simulink model "model_Quadrotor6_NonAdaptiveV2"  (R2024b)
settings: Solver=FixedStepAuto  StartTime=0.0  StopTime=T  FixedStep=0.0005  RelTol=1e-3
values from neighbouring files (symbols this model uses):
  ap1_hat = Dp/(kFF*dF*kVF^2)    (= 50.695107696)    [run_Quadrotor6_NonAdaptiveV2.m]
  ap2_hat = m*g*dcm/(kFF*dF*kVF^2)    (= 222.324678221)    [run_Quadrotor6_NonAdaptiveV2.m]
  ap3_hat = -kRT1/(kFF*dF*kVF^2)    (= -0.071301136)    [run_Quadrotor6_NonAdaptiveV2.m]
  ap4_hat = -kRT2/(kFF*dF*kVF^2)    (= -0.0008912642)    [run_Quadrotor6_NonAdaptiveV2.m]
  ay1_hat = -Dy/(kRF*dR*kVR^2)    (= -156.8624992)    [run_Quadrotor6_NonAdaptiveV2.m]
  ay2_hat = kFT1/(kRF*dR*kVR^2)    (= 0.071301136)    [run_Quadrotor6_NonAdaptiveV2.m]
  ay3_hat = kFT2/(kRF*dR*kVR^2)    (= 0.0008912642)    [run_Quadrotor6_NonAdaptiveV2.m]
  control_gains = [lambda_p lambda_y ... (first row only)    [run_Quadrotor6_NonAdaptiveV2.m]
  hp_hat = Jp/(kFF*dF*kVF^2)    (= 156.14948784)    [run_Quadrotor6_NonAdaptiveV2.m]
  hy_hat = -Jy/(kRF*dR*kVR^2)    (= -263.8142032)    [run_Quadrotor6_NonAdaptiveV2.m]
  mtr_select = 0    [run_Quadrotor6_NonAdaptiveV2.m]
  params_haaaa = [hp_hat hy_hat ... (first row only)    [run_Quadrotor6_NonAdaptiveV2.m]
settings Model: Creator=ryanmathewson  LastModifiedBy=samue
settings DebuggingCC: UnconnectedInputMsg=warning  UnconnectedOutputMsg=warning  UnconnectedLineMsg=warning
settings ModelReferenceCC: EnableRefExpFcnMdlSchedulingChecks=on
settings RTWCC: GPUComputeCapability=3.5  DLArmComputeVersion=19.05

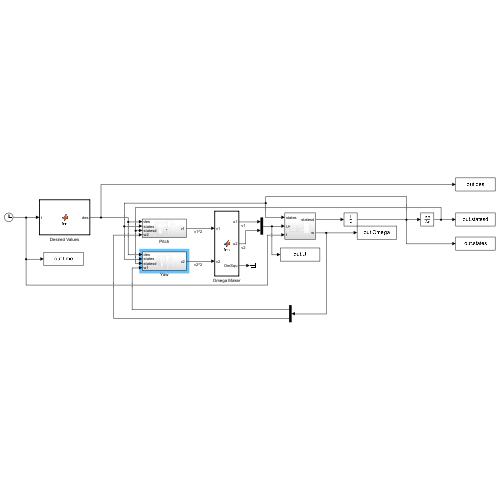
[thumbnail: Simulink's stored preview of the top-level diagram]
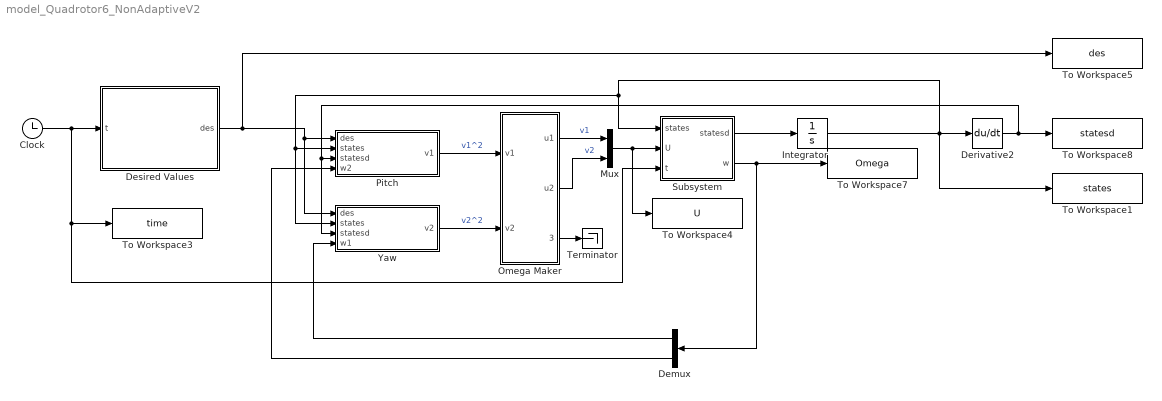
== system model_Quadrotor6_NonAdaptiveV2 ==
  Clock : Clock
  Demux : Demux  Outputs=2
  Derivative2 : Derivative
  Desired Values : MATLAB Function  TreatAsAtomicUnit=on
  Integrator : Integrator  InitialCondition=[0;0;0;0]
  Mux : Mux  Inputs=2
  Omega Maker : MATLAB Function  TreatAsAtomicUnit=on
  Pitch : Subsystem
  Subsystem : Subsystem
  Terminator : Terminator
  To Workspace1 : ToWorkspace  VariableName=states  SampleTime=-1
  To Workspace3 : ToWorkspace  VariableName=time  SampleTime=-1
  To Workspace4 : ToWorkspace  VariableName=U  SampleTime=-1
  To Workspace5 : ToWorkspace  VariableName=des  SampleTime=-1
  To Workspace7 : ToWorkspace  VariableName=Omega  SampleTime=-1
  To Workspace8 : ToWorkspace  VariableName=statesd  SampleTime=-1
  Yaw : Subsystem
  wires:
  Clock/1 -> Subsystem/3(t), To Workspace3/1, Desired Values/1(t)
  Desired Values/1(des) -> To Workspace5/1, Yaw/1(des), Pitch/1(des)
  Pitch/1(v1) -> Omega Maker/1(v1)  "v1^2"
  Yaw/1(v2) -> Omega Maker/2(v2)  "v2^2"
  Omega Maker/1(u1) -> Mux/1  "v1"
  Integrator/1 -> Derivative2/1, Yaw/2(states), Pitch/2(states), Subsystem/1(states), To Workspace1/1
  Subsystem/1(statesd) -> Integrator/1
  Derivative2/1 -> Yaw/3(statesd), Pitch/3(statesd), To Workspace8/1
  Mux/1 -> To Workspace4/1, Subsystem/2(U)
  Omega Maker/2(u2) -> Mux/2  "v2"
  Omega Maker/3(OmSqu) -> Terminator/1
  Subsystem/2(w) -> Demux/1, To Workspace7/1
  Demux/1 -> Yaw/4(w1)
  Demux/2 -> Pitch/4(w2)

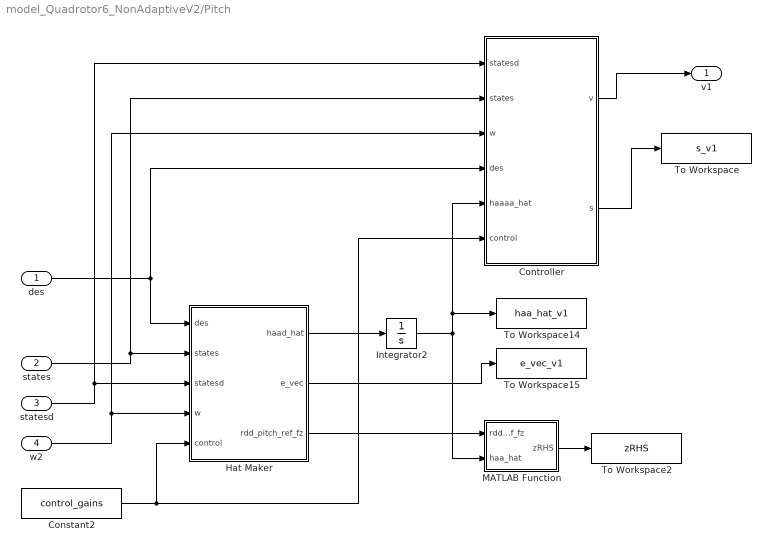
== system model_Quadrotor6_NonAdaptiveV2/Pitch ==
  des : Inport
  states : Inport  Port=2
  statesd : Inport  Port=3
  w2 : Inport  Port=4
  Constant2 : Constant  Value=control_gains
  Controller : MATLAB Function  TreatAsAtomicUnit=on
  Hat Maker : MATLAB Function  TreatAsAtomicUnit=on
  Integrator2 : Integrator  InitialCondition=[hp_hat;ap1_hat;ap2_hat;ap3_hat;ap4_hat]
  MATLAB Function : MATLAB Function  TreatAsAtomicUnit=on
  To Workspace : ToWorkspace  VariableName=s_v1  SampleTime=-1
  To Workspace14 : ToWorkspace  VariableName=haa_hat_v1  SampleTime=-1
  To Workspace15 : ToWorkspace  VariableName=e_vec_v1  SampleTime=-1
  To Workspace2 : ToWorkspace  VariableName=zRHS  SampleTime=-1
  v1 : Outport
  wires:
  Integrator2/1 -> To Workspace14/1, Controller/5(haaaa_hat), MATLAB Function/2(haa_hat)
  Hat Maker/1(haad_hat) -> Integrator2/1
  Hat Maker/2(e_vec) -> To Workspace15/1
  Controller/1(v) -> v1/1
  states/1 -> Controller/2(states), Hat Maker/2(states)
  Controller/2(s) -> To Workspace/1
  des/1 -> Hat Maker/1(des), Controller/4(des)
  statesd/1 -> Controller/1(statesd), Hat Maker/3(statesd)
  MATLAB Function/1(zRHS) -> To Workspace2/1
  Hat Maker/3(rdd_pitch_ref_fz) -> MATLAB Function/1(rdd_ref_fz)
  w2/1 -> Hat Maker/4(w), Controller/3(w)
  Constant2/1 -> Hat Maker/5(control), Controller/6(control)

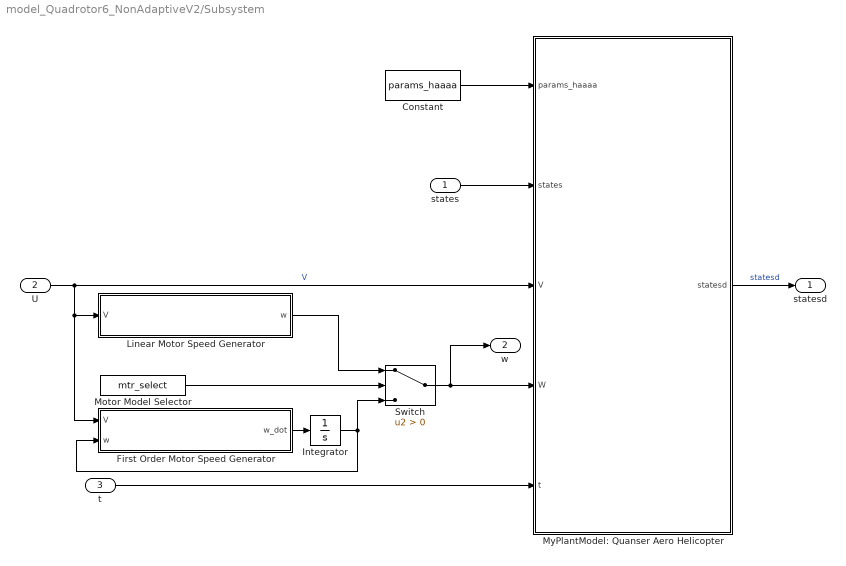
== system model_Quadrotor6_NonAdaptiveV2/Subsystem ==
  states : Inport  PortDimensions=[4 1]
  U : Inport  Port=2  PortDimensions=[2 1]
  t : Inport  Port=3
  Constant : Constant  Value=params_haaaa
  First Order Motor Speed Generator : MATLAB Function  TreatAsAtomicUnit=on
  Integrator : Integrator  InitialCondition=[0;0]
  Linear Motor Speed Generator : MATLAB Function  TreatAsAtomicUnit=on
  Motor Model Selector : Constant  Value=mtr_select
  MyPlantModel: Quanser Aero Helicopter : MATLAB Function  TreatAsAtomicUnit=on
  Switch : Switch  Criteria=u2 > Threshold  SaturateOnIntegerOverflow=off  InputSameDT=off
  statesd : Outport  PortDimensions=[4 1]
  w : Outport  Port=2  PortDimensions=[2 1]
  wires:
  states/1 -> MyPlantModel: Quanser Aero Helicopter/2(states)
  U/1 -> First Order Motor Speed Generator/1(V), Linear Motor Speed Generator/1(V), MyPlantModel: Quanser Aero Helicopter/3(V)  "V"
  t/1 -> MyPlantModel: Quanser Aero Helicopter/5(t)
  MyPlantModel: Quanser Aero Helicopter/1(statesd) -> statesd/1  "statesd"
  First Order Motor Speed Generator/1(w_dot) -> Integrator/1
  Integrator/1 -> Switch/3, First Order Motor Speed Generator/2(w)
  Constant/1 -> MyPlantModel: Quanser Aero Helicopter/1(params_haaaa)
  Switch/1 -> w/1, MyPlantModel: Quanser Aero Helicopter/4(W)
  Linear Motor Speed Generator/1(w) -> Switch/1
  Motor Model Selector/1 -> Switch/2

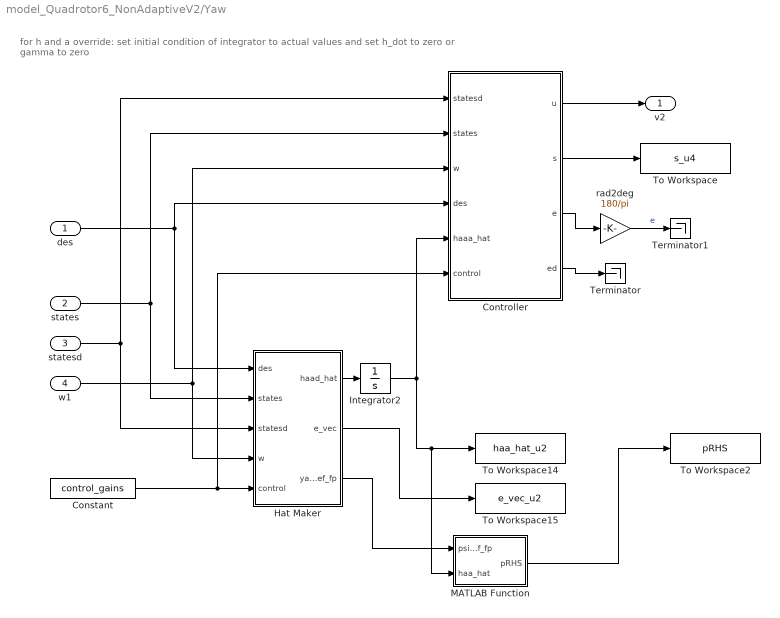
== system model_Quadrotor6_NonAdaptiveV2/Yaw ==
  note: for h and a override: set initial condition of integrator to actual values and set h_dot to zero or gamma to zero
  des : Inport
  states : Inport  Port=2
  statesd : Inport  Port=3
  w1 : Inport  Port=4
  Constant : Constant  Value=control_gains
  Controller : MATLAB Function  TreatAsAtomicUnit=on
  Hat Maker : MATLAB Function  TreatAsAtomicUnit=on
  Integrator2 : Integrator  InitialCondition=[hy_hat;ay1_hat;ay2_hat;ay3_hat]
  MATLAB Function : MATLAB Function  TreatAsAtomicUnit=on
  Terminator : Terminator
  Terminator1 : Terminator
  To Workspace : ToWorkspace  VariableName=s_u4  SampleTime=-1
  To Workspace14 : ToWorkspace  VariableName=haa_hat_u2  SampleTime=-1
  To Workspace15 : ToWorkspace  VariableName=e_vec_u2  SampleTime=-1
  To Workspace2 : ToWorkspace  VariableName=pRHS  SampleTime=-1
  rad2deg : Gain  Gain=180/pi
  v2 : Outport
  wires:
  Integrator2/1 -> Controller/5(haaa_hat), MATLAB Function/2(haa_hat), To Workspace14/1
  des/1 -> Hat Maker/1(des), Controller/4(des)
  Hat Maker/2(e_vec) -> To Workspace15/1
  Hat Maker/1(haad_hat) -> Integrator2/1
  Controller/1(u) -> v2/1
  Controller/2(s) -> To Workspace/1
  states/1 -> Controller/2(states), Hat Maker/2(states)
  statesd/1 -> Controller/1(statesd), Hat Maker/3(statesd)
  MATLAB Function/1(pRHS) -> To Workspace2/1
  Hat Maker/3(yawdd_ref_fp) -> MATLAB Function/1(psidd_ref_fp)
  w1/1 -> Hat Maker/4(w), Controller/3(w)
  Controller/3(e) -> rad2deg/1
  Controller/4(ed) -> Terminator/1
  rad2deg/1 -> Terminator1/1  "e"
  Constant/1 -> Controller/6(control), Hat Maker/5(control)

== matlab function model_Quadrotor6_NonAdaptiveV2/Yaw/Hat Maker ==
  data: des input; states input; haad_hat output; e_vec output; statesd input; yawdd_ref_fp output; w input; control input
function [haad_hat,e_vec,yawdd_ref_fp] = fcn(des,states,statesd, w, control)
%% initialize outputs
haad_hat = zeros(4,1);
e_vec = zeros(2,1);
yawdd_ref_fp = zeros(4,1);

%% separate input vectors
r_yaw = states(2,1);
r_omega_f = w;

rd_yaw = statesd(2,1);

yaw_des = des(4,1);
yawd_des = des(5,1);
yawdd_des = des(6,1);

%% parameters

gamma_0 = 0;
gamma_1 = 0;
gamma_2 = 0;
gamma_3 = 0;

lambda = control(1,2);
D = control(2,2);
eta = control(3,2);
phi_para = control(4,2);
%phi = (abs(a1v_tilde*yd + a2v_tilde*y)+eta)/(h_hat+k);

%% functions
e = r_yaw-yaw_des;
ed = rd_yaw-yawd_des;
yawdd_ref = -(-yawdd_des + lambda*ed) ; %2*lambda*ed + lambda^2*e;
s = ed + lambda*e;

%saturation function
if s>phi_para
  sat = 1;
elseif (s>=-phi_para)&&(s<=phi_para)
  sat = s/phi_para;
else
  sat = -1;
end

s_delta = s - (phi_para * sat);

f1 = rd_yaw;
f2 = r_omega_f;
f3 = sign(r_omega_f)*r_omega_f^2;

%% outputs
hd_hat  = gamma_0^2 * s_delta * (yawdd_ref + ((D + eta) * sat));
a1d_hat = -gamma_1^2 * s_delta * f1;
a2d_hat = -gamma_2^2 * s_delta * f2;
a3d_hat = -gamma_3^2 * s_delta * f3;
haad_hat = [hd_hat;a1d_hat;a2d_hat;a3d_hat];

e_vec = [e;ed];
yawdd_ref_fp = [yawdd_ref;f1;f2;f3];

== matlab function model_Quadrotor6_NonAdaptiveV2/Pitch/MATLAB Function ==
  data: rdd_ref_fz input; zRHS output; haa_hat input
function zRHS = fcn(rdd_ref_fz,haa_hat)

zRHS = transpose(haa_hat(1:5,1))*rdd_ref_fz-haa_hat(1,1);

== matlab function model_Quadrotor6_NonAdaptiveV2/Yaw/MATLAB Function ==
  data: psidd_ref_fp input; pRHS output; haa_hat input
function pRHS = fcn(psidd_ref_fp,haa_hat)

pRHS = transpose(haa_hat(1:4,1))*psidd_ref_fp;

== matlab function model_Quadrotor6_NonAdaptiveV2/Subsystem/Linear Motor Speed Generator ==
  data: V input; w output
function w = fcn(V)
% initialize output
w_dot = zeros(2,1);

% seperate input variables
V_f = V(1,1);
V_r = V(2,1);

% motor parameters
kt = 0.042219; % [N*m/A]

% linear motor relations
w_f = (1/kt)*V_f;
w_r = (1/kt)*V_r;

w = [w_f;w_r];

== matlab function model_Quadrotor6_NonAdaptiveV2/Subsystem/First Order Motor Speed Generator ==
  data: V input; w_dot output; w input
function w_dot = fcn(V, w)
% initialize output
w_dot = zeros(2,1);

% seperate input variables
V_f = V(1,1);
V_r = V(2,1);

w_f = w(1,1);
w_r = w(2,1);

% motor parameters
kt = 0.042219; % [N*m/A]
km = 0.042219; % [V/(rad/s)]
kd_f = 2.5e-7*abs(w_f) + 4.77e-06; % [N*m/(rad/s)]
kd_r = 2.5e-7*abs(w_r) + 4.77e-06; % [N*m/(rad/s)]
Rm = 8.4; % [Ohms]
Jm = 4e-6; % [kg*m^2]
Jh = 2.0160e-8; % [kg*m^2]
Jp = 4.0366e-5; % [kg*m^2]
Jeq = Jm+Jh+Jp; % [kg*m^2]

w_fdot = -(kt*km/(Rm*Jeq)+kd_f/Jeq)*w_f + (kt/(Rm*Jeq))*V_f;
w_rdot = -(kt*km/(Rm*Jeq)+kd_r/Jeq)*w_r + (kt/(Rm*Jeq))*V_r;

w_dot = [w_fdot;w_rdot];

== matlab function model_Quadrotor6_NonAdaptiveV2/Subsystem/MyPlantModel: Quanser Aero Helicopter ==
  data: params_haaaa input; states input; V input; W input; statesd output; t input
function statesd = fcn(params_haaaa, states, V, W, t)
%% initialize output
statesd = zeros(4,1);

%% seperate voltage cmd
v_fc = V(1,1);
v_rc = V(2,1);

%% seperate states
w_fs = W(1,1);
w_rs = W(2,1);
pitch = states(1,1);
pitch_dot = states(2,1);
yaw = states(3,1);
yaw_dot = states(4,1);


%% model parameters
hp = params_haaaa(1,1);
ap1 = params_haaaa(2,1);
ap2 = params_haaaa(3,1);
ap3 = params_haaaa(4,1);
ap4 = params_haaaa(5,1);

hy = params_haaaa(1,2);
ay1 = params_haaaa(2,2);
ay2 = params_haaaa(3,2);
ay3 = params_haaaa(4,2);

fp1 = pitch_dot;
fp2 = sin(pitch);
fp3 = w_rs;
fp4 = sign(w_rs)*w_rs^2;

fy1 = yaw_dot;
fy2 = w_fs;
fy3 = sign(w_fs)*w_fs^2;

%% Quanser Aero model
pitch_dotdot = -ap1/hp*fp1 -ap2/hp*fp2 -ap3/hp*fp3 -ap4/hp*fp4 ...
                              + 1/hp*sign(v_fc)*v_fc^2;

yaw_dotdot = -ay1/hy*fy1 -ay2/hy*fy2 -ay3/hy*fy3 ...
                              + 1/hy*sign(v_rc)*v_rc^2;

statesd = [pitch_dot;
           pitch_dotdot;
           yaw_dot
           yaw_dotdot];

== matlab function model_Quadrotor6_NonAdaptiveV2/Desired Values ==
  data: t input; des output
function des = fcn(t)
%% initialize outputs
des = zeros(6,1);

%% separate input vectors

%% parameters
Tp = 25;
Ty = 50;
PitchMag = deg2rad(20);
YawMag = deg2rad(30);
%% functions

% yaw_des = 0.25;
% yawd_des = 0;
% yawdd_des = 0;

yaw_des = (YawMag)*sin(2*pi*t/Ty);
yawd_des = (2*pi/Ty)*(YawMag)*cos(2*pi*t/Ty);
yawdd_des = -(2*pi/Ty)^2*(YawMag)*sin(2*pi*t/Ty);

% pitch_des = 0.25;
% pitchd_des = 0;
% pitchdd_des = 0;

pitch_des = (PitchMag)*sin(2*pi*t/Tp);
pitchd_des = (2*pi/Tp)*(PitchMag)*cos(2*pi*t/Tp);
pitchdd_des = -(2*pi/Tp)^2*(PitchMag)*sin(2*pi*t/Tp);

des = [pitch_des;
       pitchd_des;
       pitchdd_des
       yaw_des;
       yawd_des;
       yawdd_des];

== matlab function model_Quadrotor6_NonAdaptiveV2/Omega Maker ==
  data: u1 output; u2 output; v1 input; OmSqu output; v2 input
function [u1,u2,OmSqu] = fcn(v1,v2)
%% initialize outputs
u1 = 0;
u2 = 0;
OmSqu = zeros(2,1);

%% parameters
% linear motor model
kv = 1/0.0442;  % [(rad/s)/V]

%% functions
OmSqu_f = v1;
OmSqu_r = v2;

%% convert motor speed squared to control voltage
% account for square root operation on negative value
% include if statement to avoid division by zero
% use sign()

u1 = sign(OmSqu_f)*sqrt(abs(OmSqu_f));
u2 = sign(OmSqu_r)*sqrt(abs(OmSqu_r));

% if abs(OmSqu_f) < 0.01
%     u1 = OmSqu_f*(1/kv);
% else
%     u1Sign = OmSqu_f/abs(OmSqu_f);
%     u1Mag = sqrt(abs(OmSqu_f))*(1/kv);
%     u1 = u1Sign*u1Mag;
% end
% 
% if abs(OmSqu_f) < 0.01
%     u2 = OmSqu_r*(1/kv);
% else
%     u2Sign = OmSqu_r/abs(OmSqu_r);
%     u2Mag = sqrt(abs(OmSqu_r))*(1/kv);
%     u2 = u2Sign*u2Mag;
% end

%% outputs
OmSqu = [OmSqu_f;OmSqu_r]; % this is Omegas^2
% U = [u1;u2]; % this is Command Voltage

== matlab function model_Quadrotor6_NonAdaptiveV2/Pitch/Controller ==
  data: statesd input; states input; w input; des input; v output; haaaa_hat input; s output; control input
function [v,s]= fcn(statesd,states,w,des,haaaa_hat,control)
%% initialize outputs
v = zeros(1,1);
s = zeros(1,1);
baaaa = zeros(5,1);

%% separate input vectors
r_pitch = states(1,1);
r_omega_r = w;

rd_pitch = statesd(1,1);

r_pitch_des = des(1,1);
rd_pitch_des = des(2,1);
rdd_pitch_des = des(3,1);

h_hat = haaaa_hat(1,1);
a1_hat = haaaa_hat(2,1);
a2_hat = haaaa_hat(3,1);
a3_hat = haaaa_hat(4,1);
a4_hat = haaaa_hat(5,1);

%% parameters
lambda = control(1,1);
D = control(2,1);
eta = control(3,1);
phi_para = control(4,1);
% phi = (abs(a1v_tilde*yd + a2v_tilde*y)+eta)/(h_hat+k);
% g = 9.81;

%% functions
e = r_pitch-r_pitch_des;
ed = rd_pitch-rd_pitch_des;
rdd_pitch_ref = rdd_pitch_des - lambda*ed; %+ 2*lambda*ed + lambda^2*e;
s = ed + lambda*e;

if s>phi_para
  sat = 1;
elseif (s>=-phi_para)&&(s<=phi_para)
  sat = s/phi_para;
else
  sat = -1;
end

f1 = rd_pitch;
f2 = sin(r_pitch);
f3 = r_omega_r;
f4 = sign(r_omega_r)*r_omega_r^2;


% %% Override Parameters
% g = 9.81; % [m/s^2]
% m = 0.80+0.089+0.089; % [kg]
% kFF = 1.25e-6; % []
% dF = 0.2; %[m]
% dcm = 0.00325; % [m]
% Jp = 0.0219; % [kg-m^2]
% kRT1 = 1e-5; % []
% kRT2 = 1.25e-7; % []
% Dp = 0.00711; % [V-s/rad]
% 
% %% override
% h_hat = Jp/(kFF*dF);
% a1_hat = Dp/(kFF*dF);
% a2_hat = m*g*dcm/(kFF*dF);
% a3_hat = -kRT1/(kFF*dF);
% a4_hat = -kRT2/(kFF*dF);

%% outputs
v = - h_hat*(D+eta)*sat + h_hat*rdd_pitch_ref + a1_hat*f1 + a2_hat*f2 ...
                                              + a3_hat*f3 + a4_hat*f4;

== matlab function model_Quadrotor6_NonAdaptiveV2/Pitch/Hat Maker ==
  data: des input; states input; haad_hat output; e_vec output; statesd input; rdd_pitch_ref_fz output; w input; control input
function [haad_hat,e_vec,rdd_pitch_ref_fz]= fcn(des,states,statesd,w, control)
%% initialize outputs
haad_hat = zeros(5,1);
e_vec = zeros(2,1);
rdd_pitch_ref_fz = zeros(5,1);

%% separate input vectors
r_pitch = states(1,1);
r_omega_r = w;

rd_pitch = statesd(1,1);

r_pitch_des = des(1,1);
rd_pitch_des = des(2,1);
rdd_pitch_des = des(3,1);

%% parameters

gamma_0 = 0;
gamma_1 = 0;
gamma_2 = 0;
gamma_3 = 0;
gamma_4 = 0;

lambda = control(1,1);
D = control(2,1);
eta = control(3,1);
phi_para = control(4,1);
%phi = (abs(a1v_tilde*yd + a2v_tilde*y)+eta)/(h_hat+k);
g = 9.81;

%% functions
e = r_pitch-r_pitch_des;
ed = rd_pitch-rd_pitch_des;
rdd_pitch_ref = -(-rdd_pitch_des + lambda*ed); %+ 2*lambda*ed + lambda^2*e;
s = ed + lambda*e;

%saturation function
if s>phi_para
  sat = 1;
elseif (s>=-phi_para)&&(s<=phi_para)
  sat = s/phi_para;
else
  sat = -1;
end

s_delta = s - (phi_para * sat);

f1 = rd_pitch;
f2 = sin(r_pitch);
f3 = r_omega_r;
f4 = sign(r_omega_r)*r_omega_r^2;

%% outputs

hd_hat  = gamma_0^2 * s_delta * (rdd_pitch_ref + ((D + eta) * sat));
a1d_hat = -gamma_1^2 * s_delta * f1;
a2d_hat = -gamma_2^2 * s_delta * f2;
a3d_hat = -gamma_3^2 * s_delta * f3;
a4d_hat = -gamma_4^2 * s_delta * f4;
haad_hat = [hd_hat;
            a1d_hat;
            a2d_hat;
            a3d_hat;
            a4d_hat];

e_vec = [e;ed];
rdd_pitch_ref_fz = [rdd_pitch_ref;f1;f2;f3;f4];

== matlab function model_Quadrotor6_NonAdaptiveV2/Yaw/Controller ==
  data: statesd input; states input; w input; des input; u output; haaa_hat input; s output; e output; ed output; control input
function [u,s,e,ed]= fcn(statesd,states,w,des,haaa_hat, control)
%% initialize outputs
u = zeros(1,1);
s = zeros(1,1);
baaa = zeros(4,1);

%% separate input vectors
r_yaw = states(3,1);
r_omega_f = w;

rd_yaw = statesd(3,1);

yaw_des = des(4,1);
yawd_des = des(5,1);
yawdd_des = des(6,1);

h_hat = haaa_hat(1,1);
a1_hat = haaa_hat(2,1);
a2_hat = haaa_hat(3,1);
a3_hat = haaa_hat(4,1);


%% parameters
lambda = control(1,2);
D = control(2,2);
eta = control(3,2);
phi_para = control(4,2);
%phi = (abs(a1v_tilde*yd + a2v_tilde*y)+eta)/(h_hat+k);

%% functions
e = r_yaw-yaw_des;
ed = rd_yaw-yawd_des;
yawdd_ref = yawdd_des - lambda*ed; %2*lambda*ed + lambda^2*e;
s = ed + lambda*e;

if s>phi_para
  sat = 1;
elseif (s>=-phi_para)&&(s<=phi_para)
  sat = s/phi_para;
else
  sat = -1;
end

f1 = rd_yaw;
f2 = r_omega_f;
f3 = sign(r_omega_f)*r_omega_f^2;

% %% Override Parameters
% kFT1 = 1e-5; % []
% kFT2 = 1.25e-7; % []
% kRF = 1.25e-6; % []
% dR = 0.2; %[m]
% Dy = 0.0220; % [V-s/rad]
% Jy = 0.0370; % [kg-m^2]
% 
% %% Override
% h_hat = -Jy/(kRF*dR);
% a1_hat = -Dy/(kRF*dR);
% a2_hat = kFT1/(kRF*dR);
% a3_hat = kFT2/(kRF*dR);

%% outputs
u = - h_hat*(D+eta)*sat + h_hat*yawdd_ref + a1_hat*f1 + a2_hat*f2 ...
                                                      + a3_hat*f3;
